simulink model "solar"  (R2022a)
settings: Solver=VariableStepAuto  StartTime=0.0  StopTime=0.1  RelTol=1e-3
libraries: eeRmsMeasurement x4, spsSeriesRLCBranchLib x2, spsVoltageMeasurementLib x2, spsCurrentMeasurementLib x1, spsPVArrayLib x1, eePowerMeasurement x1, spspowerguiLib x1
settings Model: Creator=nikke  LastModifiedBy=nikke

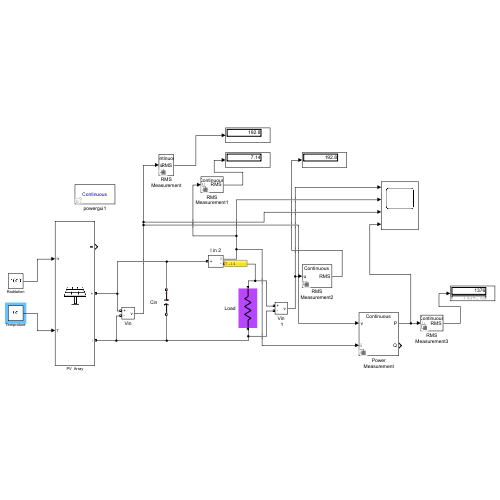
[thumbnail: Simulink's stored preview of the top-level diagram]
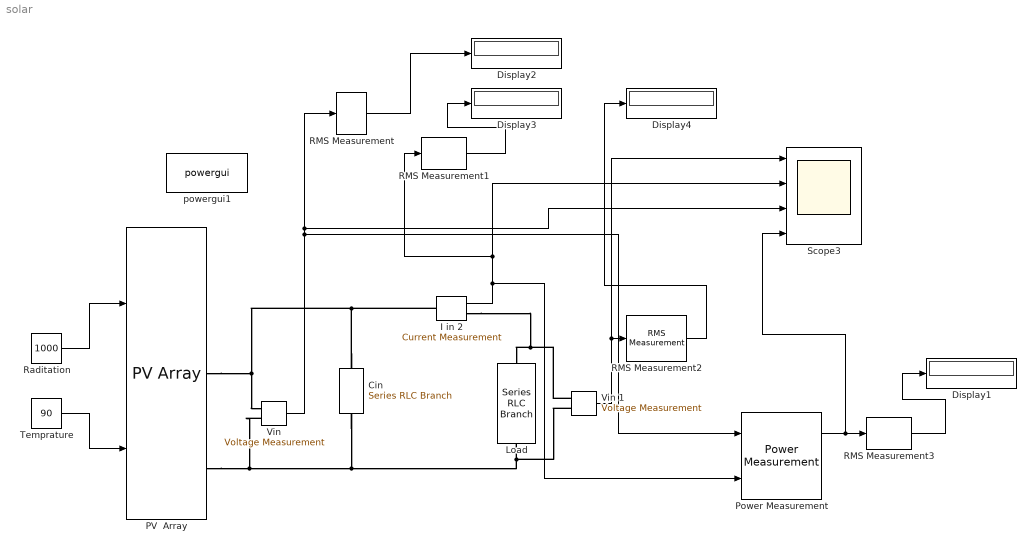
== system solar ==
  Cin : spsSeriesRLCBranchLib/Series RLC Branch  LConnTagsString=__new0  RConnTagsString=__new0  BranchType=C  Resistance=1e-4  Inductance=1e-3  SetiL0=off  InitialCurrent=0  Capacitance=200e-6  Setx0=off  InitialVoltage=0  Measurements=None
  Display{1..4} (4 alike) : Display
  I in 2 : spsCurrentMeasurementLib/Current Measurement  PhasorSimulation=off  OutputType=Complex  PSBequivalent=0
  Load : spsSeriesRLCBranchLib/Series RLC Branch  LConnTagsString=__new0  RConnTagsString=__new0  BranchType=R  Resistance=27  Inductance=1e-3  SetiL0=off  InitialCurrent=0  Capacitance=100e-6  Setx0=off  InitialVoltage=0  Measurements=None
  PV  Array : spsPVArrayLib/PV Array  Npar=2  Nser=12  PlotType=array @ 1000 W/m2 & specified temperatures  S_vec="[ 1000  500  100 ]"  Temp_C_vec="[ 45 25  ]"  ModuleName=Tata Power Solar Systems TP140SBZ  PlotWhenSelected=off  Pm=139.6944  Ncell=36  Voc=22.25  Isc=8.66  Vm=17.44  Im=8.01  beta_Voc_pc=-0.33  alpha_Isc_pc=0.063799  beta_Voc=-0.073425  alpha_Isc=0.005525  IL=8.6872  I0=9.8965e-11  nI=0.95579  Rsh=88.7762  Rs=0.27837  RobustModel=off  RobustCellTemperature=313.3991  BAL=on  Tc=1e-6  Tfilter=5e-5
  Power Measurement : eePowerMeasurement/Power Measurement  LabelModeActiveChoice=Continuous  F=60  K=[0 1 2 3]  Ts=0
      settings: SourceProductBaseCode=PS
  RMS Measurement{,1..3} (4 alike) : eeRmsMeasurement/RMS Measurement  LabelModeActiveChoice=Total  F=60  SpecifyHarmonics=off  K=[0 1 2]  Ts=0
      settings: SourceProductBaseCode=PS
  Raditation : Constant  Value=1000
  Scope3 : Scope  NumInputPorts=4
  Temprature : Constant  Value=90
  "Vin " : spsVoltageMeasurementLib/Voltage Measurement  PhasorSimulation=off  OutputType=Complex  PSBequivalent=0
  Vin 1 : spsVoltageMeasurementLib/Voltage Measurement  PhasorSimulation=off  OutputType=Complex  PSBequivalent=0
  powergui1 : spspowerguiLib/powergui  Priority=1  SimulationMode=Continuous  SampleTime=50e-6  frequency=60  Iterations=50  frequencyindice=0  Pbase=100e6  ErrMax=1e-4  UnitsV=kV  UnitsW=MW  buscounter=0  FunctionMessages=off  echomessages=off  EnableUseOfTLC=off  CurrentSourceSwitches=off  DisableSnubberDevices=off  DisableRonSwitches=off  DisableVfSwitches=off  DisplayEquations=off  AutomaticDiscreteSolvers=off  SolverType=Tustin/Backward Euler (TBE)  Interpol=off  ExternalGateDelay=off  methode=off  Ts=100  x0status=blocks  SPID=on  SwTol=0  HookPort=off  NonlinearTolerance=1e-4  nMaxIteration=100  ContinueOnMaxIteration=off  RestoreLinks=warning  ResistiveCurrentMeasurement=off  Frange=[0:2:500]  Ylog=off  Xlog=on  ShowGrid=off  save=off  variable=ZData  structure=0  ZoomFFT=off  StartTime=0.0  cycles=1  DisplayStyle=1  fundamental=60  FreqAxis=off  MaxFrequency=1000  frequencyindicesteady=1  RmsSteady=1  display=off
  wires:
  Temprature/1 -> PV  Array/2
  Raditation/1 -> PV  Array/1
  I in 2/1 -> Power Measurement/2, RMS Measurement1/1, Scope3/2
  "Vin "/1 -> Scope3/3, RMS Measurement/1, Power Measurement/1
  RMS Measurement/1 -> Display2/1
  RMS Measurement1/1 -> Display3/1
  Vin 1/1 -> Scope3/1, RMS Measurement2/1
  RMS Measurement2/1 -> Display4/1
  Power Measurement/1 -> Scope3/4, RMS Measurement3/1
  RMS Measurement3/1 -> Display1/1
  connections:
  PV  Array/RConn2 -- "Vin "/LConn2 -- Cin/RConn1 -- Vin 1/LConn2 -- Load/RConn1
  Vin 1/LConn1 -- I in 2/RConn1 -- Load/LConn1
  PV  Array/RConn1 -- I in 2/LConn1 -- Cin/LConn1 -- "Vin "/LConn1
